simulink model "Controllo_2_2"  (Simulink 7.8)
settings: Solver=ode23s  StartTime=0.0  StopTime=250  RelTol=1e-10
libraries: simulink x2
settings Model: Creator=dAnIeLe  LastModifiedBy=dAnIeLe
settings DebuggingCC: SolverPrmCheckMsg=none

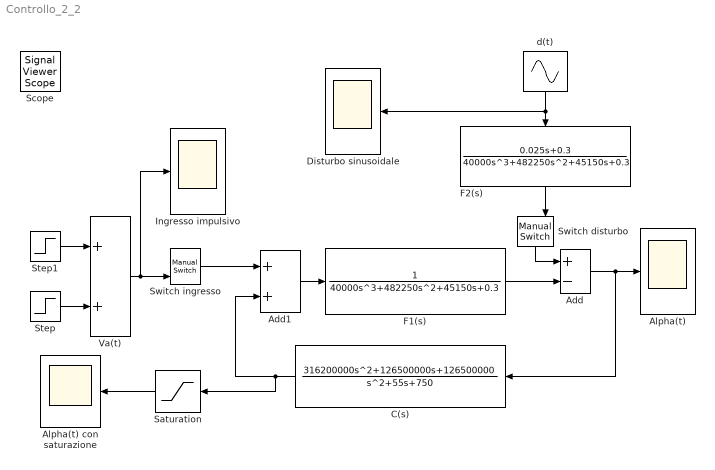
== system Controllo_2_2 ==
  Add : Sum  Inputs=+-
  Add1 : Sum
  Alpha(t) : Scope
      settings: TimeRange=15  YMin=-9e-06  YMax=9.999999999999989e-07
  Alpha(t) con saturazione : Scope
      settings: TimeRange=30  YMin=-0.5236  YMax=-0.5236  SaveName=ScopeData2
  C(s) : TransferFcn  Numerator=[316200000 126500000 126500000]  Denominator=[1 55 750]
  Disturbo sinusoidale : Scope
      settings: TimeRange=7  YMin=0.95  YMax=1.05  SaveName=ScopeData3
  F1(s) : TransferFcn  Denominator=[40000 482250 45150 0.3]
  F2(s) : TransferFcn  Numerator=[0.025 0.3]  Denominator=[40000 482250 45150 0.3]
  Ingresso impulsivo : Scope
      settings: TimeRange=7  YMin=0.95  YMax=1.05
  Saturation : Saturate  UpperLimit=0.5236  LowerLimit=-0.5236
  Step : Step  Time=0  SampleTime=0
  Step1 : Step  Time=0.5  Before=1  After=0  SampleTime=0
  Switch disturbo : simulink/Signal Routing/Manual Switch  sw=1  action=0  varsize=off
  Switch ingresso : simulink/Signal Routing/Manual Switch  sw=0  action=0  varsize=off
  Va(t) : Sum
  d(t) : Sin  Amplitude=100  Frequency=0.628  SampleTime=0
  Scope : SignalViewerScope  IOType=viewer  RefreshTime=0.035000
  wires:
  d(t)/1 -> F2(s)/1, Disturbo sinusoidale/1
  F1(s)/1 -> Add/2
  Add/1 -> C(s)/1, Alpha(t)/1
  C(s)/1 -> Add1/2, Saturation/1
  Add1/1 -> F1(s)/1
  Step1/1 -> Va(t)/1
  Step/1 -> Va(t)/2
  Switch disturbo/1 -> Add/1
  F2(s)/1 -> Switch disturbo/2
  Switch ingresso/1 -> Add1/1
  Va(t)/1 -> Switch ingresso/2, Ingresso impulsivo/1
  Saturation/1 -> Alpha(t) con saturazione/1
